simulink model "sim3d"  (R2020a)
settings: Solver=VariableStepAuto  StartTime=0.0  StopTime=T  RelTol=1e-3
StopFcn:
  | save_3DSim_data
values from neighbouring files (symbols this model uses):
  IMUALIGNMENT = eul2rotm([-pi, 0, 0])    [setImuParameters.m]
  refDirections = ones(numPoses,1)    [simulate_3D_scenario.m]
  refPath = refPoses{1,1}    [select_waypoints.m]
undefined symbols (not defined in the file or in its folder): frontBumper_lidarSpecs, rearBumper_lidarSpecs
libraries: simulink_extras x3, drivingvehiclecontroller x2, drivinglib x2, sim3dphyssensorlib x2, autolibshared x1, sim3dautolib x1, mspsensorlib x1, sim3dlib x1
settings Model: Creator=sjur_  LastModifiedBy=sjurgw

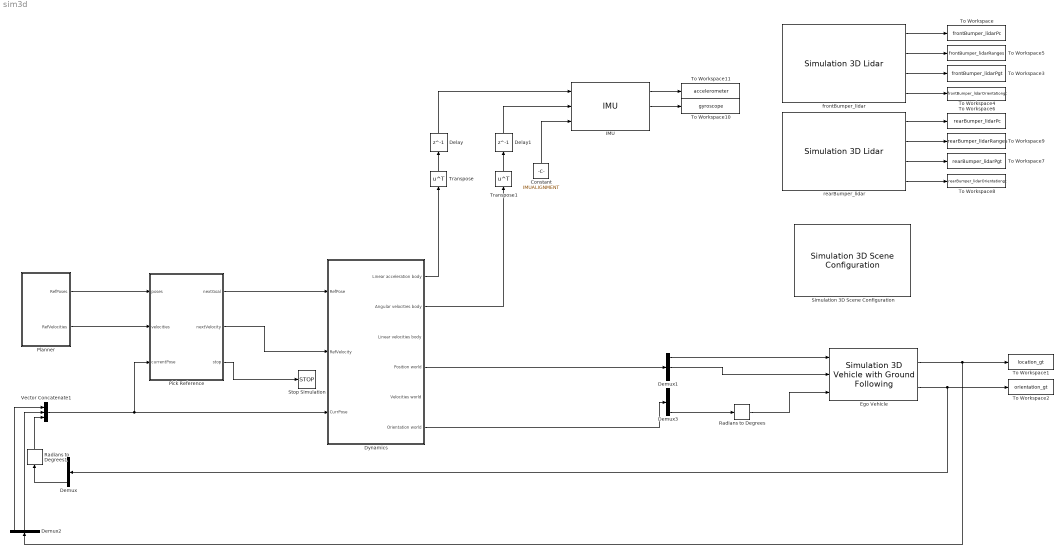
== system sim3d ==
  Constant : Constant  Value=IMUALIGNMENT
  Delay : Delay  DelayLength=1
  Delay1 : Delay  DelayLength=1
  Demux{,1..3} (4 alike) : Demux  Outputs=3
  Dynamics : Subsystem
  Ego Vehicle : sim3dautolib/Simulation 3D Vehicle with Ground Following  Priority=-1  PassVehMesh=Box truck  VehColor=Red  InitialPos=[0, 0, 0]  InitialRot=[0, 0, 0]  ActorName=EgoVehicle  SampleTime=-1  ActorType=SimulinkVehicle  ID=C  aMode=3  ActorTag=EgoVehicle  CoordinateScheme=ISO  TransformOutportEnabled=on
      settings: SourceProductBaseCode=DR,VE
  IMU : mspsensorlib/IMU  DispRefFrame=NED  Temperature=25  MagneticFieldNED=[ 27.5550, -2.4169, -16.0849 ]  MagneticFieldENU=[ -2.4169, 27.5550, 16.0849 ]  SeedDouble=67  SimulateUsing=Interpreted execution  AccelParamsMeasurementRange=Inf  AccelParamsResolution=imuParams.acc_resolution  AccelParamsConstantBias=imuParams.acc_constantBias  AccelParamsAxesMisalignment=[ 0, 0, 0 ]  AccelParamsNoiseDensity=imuParams.acc_velocity_randomWalk  AccelParamsBiasInstability=imuParams.acc_biasInstability  AccelParamsRandomWalk=imuParams.acc_acceleration_randomWalk  AccelParamsTemperatureBias=[ 0, 0, 0 ]  AccelParamsTemperatureScaleFactor=[ 0, 0, 0 ]  GyroParamsMeasurementRange=Inf  GyroParamsResolution=imuParams.gyro_resolution  GyroParamsConstantBias=imuParams.gyro_constantBias  GyroParamsAxesMisalignment=[ 0, 0, 0 ]  GyroParamsAccelerationBias=imuParams.gyro_accelerationBias  GyroParamsNoiseDensity=imuParams.gyro_angle_randomWalk  GyroParamsBiasInstability=imuParams.gyro_biasInstability  GyroParamsRandomWalk=imuParams.gyro_rate_randomWalk  GyroParamsTemperatureBias=[ 0, 0, 0 ]  GyroParamsTemperatureScaleFactor=[ 0, 0, 0 ]  MagParamsMeasurementRange=Inf  MagParamsResolution=0  MagParamsConstantBias=[ 0, 0, 0 ]  MagParamsAxesMisalignment=[ 0, 0, 0 ]  MagParamsNoiseDensity=[ 0, 0, 0 ]  MagParamsBiasInstability=[ 0, 0, 0 ]  MagParamsRandomWalk=[ 0, 0, 0 ]  MagParamsTemperatureBias=[ 0, 0, 0 ]  MagParamsTemperatureScaleFactor=[ 0, 0, 0 ]
      settings: SourceProductBaseCode=TF,NV
  Pick Reference : MATLAB Function  TreatAsAtomicUnit=on
  Planner : Subsystem
  Radians to Degrees : simulink_extras/Transformations/Radians to Degrees
  Radians to Degrees1 : simulink_extras/Transformations/Radians to Degrees
  Simulation 3D Scene Configuration : sim3dlib/Simulation 3D Scene Configuration  Priority=0  ProjectFormat=Unreal Editor  SceneDesc=Straight road  ProjectName=VehicleSimulation.exe  ScenePath=/Game/Maps/HwStrght  UEProjPath=C:\Local\SimpleTunnel\Tunnel.uproject  vehTagList={'EgoVehicle';'Scene Origin'}  vehTag=EgoVehicle  OpVisEn=off  Ts=1/60  EnableWindow=on  sensorTag=MainCamera1  sensorId=1  sensorName=MainCamera1  mountLoc=Origin  offsetFlag=off  tmountOffset=[0, 0, 0]  rmountOffset=[0, 0, 0]  HorizontalResolution=1280  VerticalResolution=720  HorizontalFOV=60  mountPoint=[0 0 0]  mountOrientation=[0 0 0]  aMode=3  ID=1
      settings: SourceProductBaseCode=DR,VE
  Stop Simulation : Stop
  To Workspace : ToWorkspace  VariableName=frontBumper_lidarPc  SaveFormat=Structure With Time  SampleTime=-1
  To Workspace1 : ToWorkspace  VariableName=location_gt  SaveFormat=Structure With Time  SampleTime=-1
  To Workspace10 : ToWorkspace  VariableName=gyroscope  SaveFormat=Structure With Time  SampleTime=-1
  To Workspace11 : ToWorkspace  VariableName=accelerometer  SaveFormat=Structure With Time  SampleTime=-1
  To Workspace2 : ToWorkspace  VariableName=orientation_gt  SaveFormat=Structure With Time  SampleTime=-1
  To Workspace3 : ToWorkspace  VariableName=frontBumper_lidarPgt  SaveFormat=Structure With Time  SampleTime=-1
  To Workspace4 : ToWorkspace  VariableName=frontBumper_lidarOrientationgt  SaveFormat=Structure With Time  SampleTime=-1
  To Workspace5 : ToWorkspace  VariableName=frontBumper_lidarRanges  SaveFormat=Structure With Time  SampleTime=-1
  To Workspace6 : ToWorkspace  VariableName=rearBumper_lidarPc  SaveFormat=Structure With Time  SampleTime=-1
  To Workspace7 : ToWorkspace  VariableName=rearBumper_lidarPgt  SaveFormat=Structure With Time  SampleTime=-1
  To Workspace8 : ToWorkspace  VariableName=rearBumper_lidarOrientationgt  SaveFormat=Structure With Time  SampleTime=-1
  To Workspace9 : ToWorkspace  VariableName=rearBumper_lidarRanges  SaveFormat=Structure With Time  SampleTime=-1
  Transpose : Math  Operator=transpose  SaturateOnIntegerOverflow=on
  Transpose1 : Math  Operator=transpose  SaturateOnIntegerOverflow=on
  Vector Concatenate1 : Concatenate  NumInputs=3
  frontBumper_lidar : sim3dphyssensorlib/Simulation 3D Lidar  Priority=1  sensorTag=Sim3dSensor1  sensorId=1  sensorName=Sim3dSensor1  vehTagList={'EgoVehicle';'Scene Origin'}  vehTag=EgoVehicle  mountLoc=Front bumper  offsetFlag=on  tmountOffset=[0.5, 0, -0.1]  rmountOffset=[0, 0, 0]  DetectionRange=frontBumper_lidarSpecs.detectionRange  RangeResolution=frontBumper_lidarSpecs.rangeResolution  VerticalFOV=frontBumper_lidarSpecs.verticalFOV  VerticalResolution=frontBumper_lidarSpecs.verticalResolution  HorizontalFOV=frontBumper_lidarSpecs.horizontalFOV  HorizontalResolution=frontBumper_lidarSpecs.horizontalResolution  DistanceOutportEnabled=on  TransformOutportEnabled=on  SampleTime=1/frontBumper_lidarSpecs.frequency  mountPoint=[5.59999990463257 0 0.5]  mountOrientation=[0 0 0]  aMode=3  ID=1
      settings: SourceProductBaseCode=DR,VE
  rearBumper_lidar : sim3dphyssensorlib/Simulation 3D Lidar  Priority=1  sensorTag=Sim3dSensor2  sensorId=2  sensorName=Sim3dSensor2  vehTagList={'EgoVehicle';'Scene Origin'}  vehTag=EgoVehicle  mountLoc=Rear bumper  offsetFlag=on  tmountOffset=[0.5, 0, -0.1]  rmountOffset=[0, 0, 0]  DetectionRange=rearBumper_lidarSpecs.detectionRange  RangeResolution=rearBumper_lidarSpecs.rangeResolution  VerticalFOV=rearBumper_lidarSpecs.verticalFOV  VerticalResolution=rearBumper_lidarSpecs.verticalResolution  HorizontalFOV=rearBumper_lidarSpecs.horizontalFOV  HorizontalResolution=rearBumper_lidarSpecs.horizontalResolution  DistanceOutportEnabled=on  TransformOutportEnabled=on  SampleTime=1/rearBumper_lidarSpecs.frequency  mountPoint=[-4.5 0 0.5]  mountOrientation=[0 0 180]  aMode=3  ID=2
      settings: SourceProductBaseCode=DR,VE
  wires:
  frontBumper_lidar/1 -> To Workspace/1
  rearBumper_lidar/4 -> To Workspace8/1
  rearBumper_lidar/1 -> To Workspace6/1
  rearBumper_lidar/2 -> To Workspace9/1
  rearBumper_lidar/3 -> To Workspace7/1
  frontBumper_lidar/2 -> To Workspace5/1
  frontBumper_lidar/3 -> To Workspace3/1
  frontBumper_lidar/4 -> To Workspace4/1
  Demux2/2 -> Vector Concatenate1/2
  Demux/3 -> Radians to Degrees1/1
  Ego Vehicle/1 -> To Workspace1/1, Demux2/1
  Ego Vehicle/2 -> To Workspace2/1, Demux/1
  Dynamics/4(Position world) -> Demux1/1
  Demux1/1 -> Ego Vehicle/1
  Demux1/2 -> Ego Vehicle/2
  Dynamics/6(Orientation world) -> Demux3/1
  Demux3/3 -> Radians to Degrees/1
  Radians to Degrees/1 -> Ego Vehicle/3
  Demux2/1 -> Vector Concatenate1/1
  Vector Concatenate1/1 -> Pick Reference/3(currentPose), Dynamics/3(CurrPose)
  Planner/2(RefVelocities) -> Pick Reference/2(velocities)
  Planner/1(RefPoses) -> Pick Reference/1(poses)
  Pick Reference/2(nextVelocity) -> Dynamics/2(RefVelocity)
  Pick Reference/1(nextGoal) -> Dynamics/1(RefPose)
  Radians to Degrees1/1 -> Vector Concatenate1/3
  Dynamics/1(Linear acceleration body) -> Transpose/1
  Dynamics/2(Angular velocities body) -> Transpose1/1
  Transpose/1 -> Delay/1
  Transpose1/1 -> Delay1/1
  Delay/1 -> IMU/1
  Delay1/1 -> IMU/2
  IMU/1 -> To Workspace11/1
  IMU/2 -> To Workspace10/1
  Constant/1 -> IMU/3
  Pick Reference/3(stop) -> Stop Simulation/1

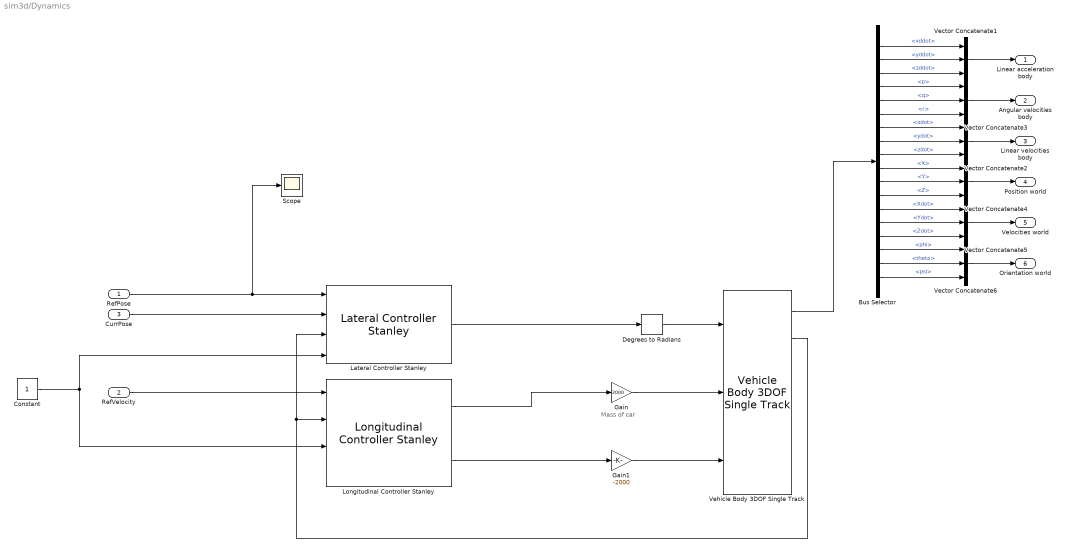
== system sim3d/Dynamics ==
  note: Mass of car
  RefPose : Inport
  RefVelocity : Inport  Port=2
  CurrPose : Inport  Port=3
  Bus Selector : BusSelector  OutputSignals=BdyFrm.Cg.Acc.xddot,BdyFrm.Cg.Acc.yddot,BdyFrm.Cg.Acc.zddot,BdyFrm.Cg.AngVel.p,BdyFrm.Cg.AngVel.q,BdyFrm.Cg.AngVel.r,BdyFrm.Cg.Vel.xdot,BdyFrm.Cg.Vel.ydot,BdyFrm.Cg.Vel.zdot,InertFrm.Cg.Disp.X,InertFrm.Cg.Disp.Y,InertFrm.Cg.Disp.Z,InertFrm.Cg.Vel.Xdot,InertFrm.Cg.Vel.Ydot,InertFrm.Cg.Vel.Zdot,InertFrm.Cg.Ang.phi,InertFrm.Cg.Ang.theta,InertFrm.Cg.Ang.psi
  Constant : Constant
  Degrees to Radians : simulink_extras/Transformations/Degrees to Radians
  Gain : Gain  Gain=2000
  Gain1 : Gain  Gain=-2000
  Lateral Controller Stanley : drivingvehiclecontroller/Lateral Controller Stanley  ModelType=Kinematic bicycle model  PositionGainF=2.5  PositionGainR=2.5  YawRateGain=0.2  DelayGain=0.2  VehicleMass=1575  Lf=1.2  Lr=1.6  TireStiffness=19000  Wheelbase=2.8  MaxSteeringAngle=35
      settings: SourceProductBaseCode=DR
  Longitudinal Controller Stanley : drivingvehiclecontroller/Longitudinal Controller Stanley  Kp=2.5  Ki=1  SampleTime=0.05  MaxAcceleration=1.5  MaxDeceleration=6
      settings: SourceProductBaseCode=DR
  Scope : Scope
  Vector Concatenate{1..6} (6 alike) : Concatenate  NumInputs=3
  Vehicle Body 3DOF Single Track : autolibshared/Vehicle Body 3DOF Single Track  trackMode=Single (bicycle)  inputMode=External longitudinal forces  frontSteerMode=on  rearSteerMode=off  windMode=off  muMode=off  extFMode=off  extMMode=off  extXo=off  extpsio=off  extxdoto=off  extro=off  extYo=off  extTamb=off  extydoto=off  aMode=2  NF=2  NR=2  m=2000  a=1.4  b=1.6  h=0.35  X_o=0  xdot_o=0  CalphaMode=off  sigmaMode=on  d=0  w=[1.4,1.4]  Cy_f=12e3  Cy_r=11e3  sigma_f=.1  sigma_r=.1  alpha_f_brk=[-.1 .1]  Cy_f_data=[-9e3 9e3]  alpha_r_brk=[-.1 .1]  Cy_r_data=[-9e3 9e3]  Y_o=0  ydot_o=0  Izz=4000  psi_o=0  r_o=0  Af=2  Cd=.3  Cl=.1  Cpm=.1  beta_w=[0:0.01:0.3]  Cs=[0:0.03:0.9]  Cym=[0:0.01:0.3]  Pabs=101325  Tair=273  g=9.81  mu=1  xdot_tol=.01  Fznom=5000  Fxtire_sat=7e4  Fytire_sat=7e4  longOff=0  latOff=0  vertOff=0  wrapAng=off
      settings: SourceProductBaseCode=PW,MT,VE,VP
  Linear acceleration body : Outport
  Angular velocities body : Outport  Port=2
  Linear velocities body : Outport  Port=3
  Position world : Outport  Port=4
  Velocities world : Outport  Port=5
  Orientation world : Outport  Port=6
  wires:
  RefVelocity/1 -> Longitudinal Controller Stanley/1
  CurrPose/1 -> Lateral Controller Stanley/2
  Constant/1 -> Lateral Controller Stanley/4, Longitudinal Controller Stanley/3
  Longitudinal Controller Stanley/1 -> Gain/1
  Longitudinal Controller Stanley/2 -> Gain1/1
  Bus Selector/1 -> Vector Concatenate1/1  "<xddot>"
  Bus Selector/2 -> Vector Concatenate1/2  "<yddot>"
  Bus Selector/3 -> Vector Concatenate1/3  "<zddot>"
  Vector Concatenate1/1 -> Linear acceleration body/1
  Bus Selector/4 -> Vector Concatenate3/1  "<p>"
  Bus Selector/5 -> Vector Concatenate3/2  "<q>"
  Bus Selector/6 -> Vector Concatenate3/3  "<r>"
  Vector Concatenate3/1 -> Angular velocities body/1
  Vector Concatenate2/1 -> Linear velocities body/1
  Bus Selector/7 -> Vector Concatenate2/1  "<xdot>"
  Bus Selector/8 -> Vector Concatenate2/2  "<ydot>"
  Bus Selector/9 -> Vector Concatenate2/3  "<zdot>"
  Bus Selector/10 -> Vector Concatenate4/1  "<X>"
  Bus Selector/11 -> Vector Concatenate4/2  "<Y>"
  Bus Selector/12 -> Vector Concatenate4/3  "<Z>"
  Vector Concatenate4/1 -> Position world/1
  Vector Concatenate5/1 -> Velocities world/1
  Bus Selector/13 -> Vector Concatenate5/1  "<Xdot>"
  Bus Selector/14 -> Vector Concatenate5/2  "<Ydot>"
  Bus Selector/15 -> Vector Concatenate5/3  "<Zdot>"
  Vector Concatenate6/1 -> Orientation world/1
  Bus Selector/16 -> Vector Concatenate6/1  "<phi>"
  Bus Selector/17 -> Vector Concatenate6/2  "<theta>"
  Bus Selector/18 -> Vector Concatenate6/3  "<psi>"
  RefPose/1 -> Scope/1, Lateral Controller Stanley/1
  ? -> ?
  Lateral Controller Stanley/1 -> Degrees to Radians/1
  Vehicle Body 3DOF Single Track/1 -> Bus Selector/1
  Vehicle Body 3DOF Single Track/2 -> Lateral Controller Stanley/3, Longitudinal Controller Stanley/2
  Degrees to Radians/1 -> Vehicle Body 3DOF Single Track/1
  Gain/1 -> Vehicle Body 3DOF Single Track/2
  Gain1/1 -> Vehicle Body 3DOF Single Track/3

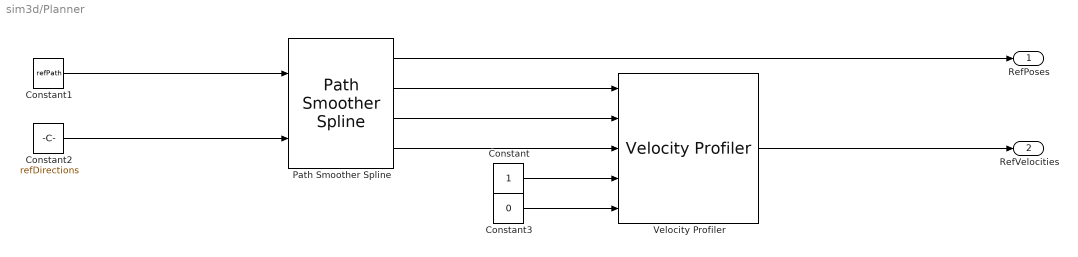
== system sim3d/Planner ==
  Constant : Constant
  Constant1 : Constant  Value=refPath
  Constant2 : Constant  Value=refDirections
  Constant3 : Constant  Value=0
  Path Smoother Spline : drivinglib/Path Smoother Spline  NumSmoothPoses=50  MinSeparation=1e-3  SampleTime=0.5  ShowOptionalOutports=on  SimulateUsing=Code generation
      settings: SourceProductBaseCode=DR
  Velocity Profiler : drivinglib/Velocity Profiler  MaxLongitudinalAccel=3  MaxLongitudinalDecel=6  MaxSpeed=6  MaxLongitudinalJerk=1  MaxLateralAccel=1  ShowOptionalOutport=off  SampleTime=-1  SimulateUsing=Code generation
      settings: SourceProductBaseCode=DR
  RefPoses : Outport
  RefVelocities : Outport  Port=2
  wires:
  Path Smoother Spline/4 -> Velocity Profiler/3
  Path Smoother Spline/3 -> Velocity Profiler/2
  Path Smoother Spline/2 -> Velocity Profiler/1
  Constant1/1 -> Path Smoother Spline/1
  Path Smoother Spline/1 -> RefPoses/1
  Constant2/1 -> Path Smoother Spline/2
  Velocity Profiler/1 -> RefVelocities/1
  Constant/1 -> Velocity Profiler/4
  Constant3/1 -> Velocity Profiler/5

== matlab function sim3d/Pick Reference ==
  data: poses input; nextGoal output size=[1,3]; velocities input; nextVelocity output size=1; currentPose input; stop output
function [nextGoal, nextVelocity, stop]= ReferencePicker(poses, velocities, currentPose)
persistent idx;

if isempty(idx)
    idx = 1;
end
stop = 0;
currentRefPose = poses(idx,:);
distTol = 1;
dist = sqrt((currentRefPose(1) - currentPose(1))^2 + (currentRefPose(2) - currentPose(2))^2);

if dist <= distTol
    if idx+1 >= size(poses, 1)
        stop = 1;
    else
        idx = idx + 1;
    end
end
targetRadians = poses(idx, 3)*pi/180;
targetRadians = targetRadians - 2*pi*floor( (targetRadians+pi)/(2*pi) ); 
targetAngle = targetRadians * 180/pi;
nextGoal = [poses(idx, 1), poses(idx,2), targetAngle];
nextVelocity = velocities(idx);
